simulink library "three_phase_voltage_with_frt_emulator"  (R2026a)
settings: Solver=VariableStepAuto
undefined symbols (not defined in the file): filters, frt_data, grid_emu, start_time_LVRT
libraries: $bdroot x6
settings Model: Creator=dbagn  LastModifiedBy=ltnbda

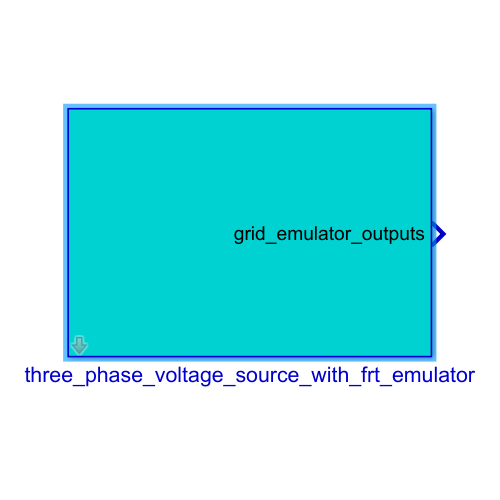
[thumbnail: Simulink's stored preview of the top-level diagram]
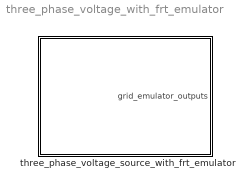
== system three_phase_voltage_with_frt_emulator ==
  three_phase_voltage_source_with_frt_emulator : Subsystem  mask{nominal_frequency_m=grid_emu.fgrid_nom, nominal_voltage_m=grid_emu.us_secondary_nom, Vemu_ref_norm_m=grid_emu.Vemu_ref_norm, vp_xi_pu_m=grid_emu.up_xi_pu_ref, vp_eta_pu_m=grid_emu.up_eta_pu_ref, vn_xi_pu_m=grid_emu.un_xi_pu_ref, vn_eta_pu_m=grid_emu.un_eta_pu, Am=filters.afe.SOF_50Hz.ss_c.A, Bm=filters.afe.SOF_50Hz.ss_c.B, Cm=filters.afe.SOF_50Hz.ss_c.C, enable_frt_1_m=frt_data.enable_frt_1, enable_frt_2_m=frt_data.enable_frt_2, start_time_LVRT_m=frt_data.start_time_LVRT, end_time_LVRT_m=frt_data.end_time_LVRT, deepPOSxi_m=frt_data.deepPOSxi, deepPOSeta_m=frt_data.deepPOSeta, deepNEGxi_m=frt_data.deepNEGxi, deepNEGeta_m=frt_data.deepNEGeta, Amplitude_U_m=frt_data.Amplitude_U, Amplitude_V_m=frt_data.Amplitude_V, Amplitude_W_m=frt_data.Amplitude_W, t_ramp_m=frt_data.t_ramp, Phase_shift_m=frt_data.Phase_shift}
      mask prompts: nominal_frequency_m "Nominal Frequency [Hz]"; nominal_voltage_m "Nominal Voltage [V]"; Vemu_ref_norm_m "Vemu_ref_norm"; vp_xi_pu_m "Vp_xi_pu [pu]"; vp_eta_pu_m "Vp_eta_pu [pu]"; vn_xi_pu_m "Vn_xi_pu [pu]"; vn_eta_pu_m "Vn_eta_pu [pu]"; Am "LVRT_flt_ss.A"; Bm "LVRT_flt_ss.B"; Cm "LVRT_flt_ss.C"; enable_frt_1_m "enable_frt_1"; enable_frt_2_m "enable_frt_2"; start_time_LVRT_m "Start_time_LVRT"; end_time_LVRT_m "End_time_LVRT"; deepPOSxi_m "deepPOSxi"; deepPOSeta_m "deepPOSeta"; deepNEGxi_m "deepNEGxi"; deepNEGeta_m "deepNEGeta"; Amplitude_U_m "Amplitude_U"; Amplitude_V_m "Amplitude_V"; Amplitude_W_m "Amplitude_W"; t_ramp_m "t_ramp"; Phase_shift_m "Phase_shift"

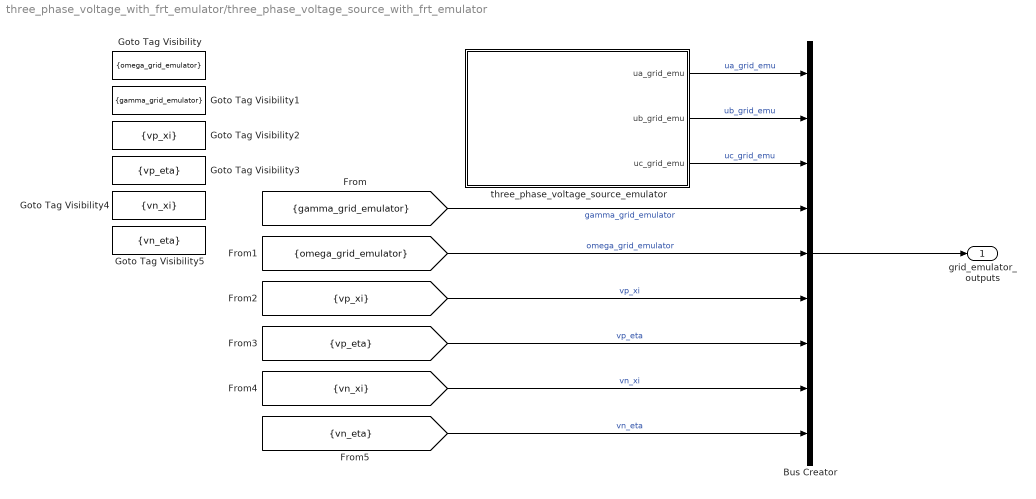
== system three_phase_voltage_with_frt_emulator/three_phase_voltage_source_with_frt_emulator ==
  Bus Creator : BusCreator  Inputs=9
  Goto Tag Visibility : GotoTagVisibility  GotoTag=omega_grid_emulator
  Goto Tag Visibility1 : GotoTagVisibility  GotoTag=gamma_grid_emulator
  Goto Tag Visibility2 : GotoTagVisibility  GotoTag=vp_xi
  Goto Tag Visibility3 : GotoTagVisibility  GotoTag=vp_eta
  Goto Tag Visibility4 : GotoTagVisibility  GotoTag=vn_xi
  Goto Tag Visibility5 : GotoTagVisibility  GotoTag=vn_eta
  three_phase_voltage_source_emulator : Subsystem
  grid_emulator_outputs : Outport  VectorParamsAs1DForOutWhenUnconnected=off
  wires:
  Bus Creator/1 -> grid_emulator_outputs/1
  three_phase_voltage_source_emulator/1(ua_grid_emu) -> Bus Creator/1  "ua_grid_emu"
  three_phase_voltage_source_emulator/2(ub_grid_emu) -> Bus Creator/2  "ub_grid_emu"
  three_phase_voltage_source_emulator/3(uc_grid_emu) -> Bus Creator/3  "uc_grid_emu"
  [omega_grid_emulator] -> Bus Creator/5  "omega_grid_emulator"
  [gamma_grid_emulator] -> Bus Creator/4  "gamma_grid_emulator"
  [vp_xi] -> Bus Creator/6  "vp_xi"
  [vp_eta] -> Bus Creator/7  "vp_eta"
  [vn_xi] -> Bus Creator/8  "vn_xi"
  [vn_eta] -> Bus Creator/9  "vn_eta"

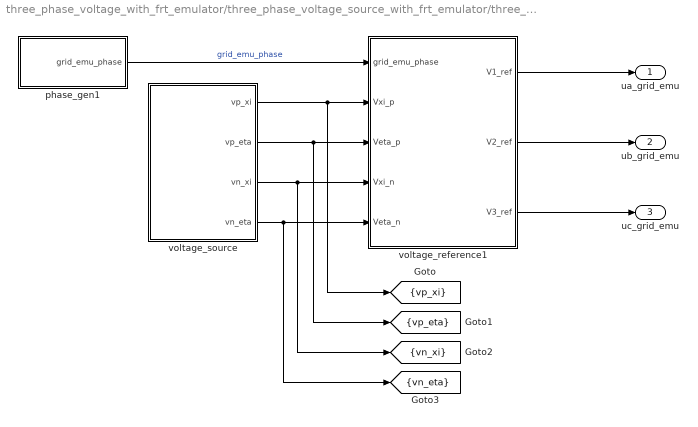
== system three_phase_voltage_with_frt_emulator/three_phase_voltage_source_with_frt_emulator/three_phase_voltage_source_emulator ==
  phase_gen1 : Subsystem
  voltage_reference1 : Subsystem
  voltage_source : Subsystem
  ua_grid_emu : Outport  VectorParamsAs1DForOutWhenUnconnected=off
  ub_grid_emu : Outport  Port=2  VectorParamsAs1DForOutWhenUnconnected=off
  uc_grid_emu : Outport  Port=3  VectorParamsAs1DForOutWhenUnconnected=off
  tag scope: vn_eta=scoped, vn_xi=scoped, vp_eta=scoped, vp_xi=scoped
  wires:
  voltage_reference1/2(V2_ref) -> ub_grid_emu/1
  voltage_reference1/3(V3_ref) -> uc_grid_emu/1
  voltage_source/3(vn_xi) -> [vn_xi], voltage_reference1/4(Vxi_n)
  voltage_source/1(vp_xi) -> [vp_xi], voltage_reference1/2(Vxi_p)
  voltage_source/4(vn_eta) -> [vn_eta], voltage_reference1/5(Veta_n)
  phase_gen1/1(grid_emu_phase) -> voltage_reference1/1(grid_emu_phase)  "grid_emu_phase"
  voltage_reference1/1(V1_ref) -> ua_grid_emu/1
  voltage_source/2(vp_eta) -> [vp_eta], voltage_reference1/3(Veta_p)

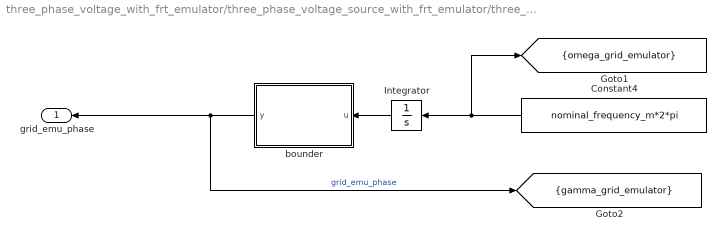
== system three_phase_voltage_with_frt_emulator/three_phase_voltage_source_with_frt_emulator/three_phase_voltage_source_emulator/phase_gen1 ==
  Constant4 : Constant  Value=nominal_frequency_m*2*pi
  Integrator : Integrator
  bounder : MATLAB Function  TreatAsAtomicUnit=on
  grid_emu_phase : Outport  VectorParamsAs1DForOutWhenUnconnected=off
  tag scope: gamma_grid_emulator=scoped, omega_grid_emulator=scoped
  wires:
  Integrator/1 -> bounder/1(u)
  Constant4/1 -> Integrator/1, [omega_grid_emulator]
  bounder/1(y) -> grid_emu_phase/1, [gamma_grid_emulator]  "grid_emu_phase"

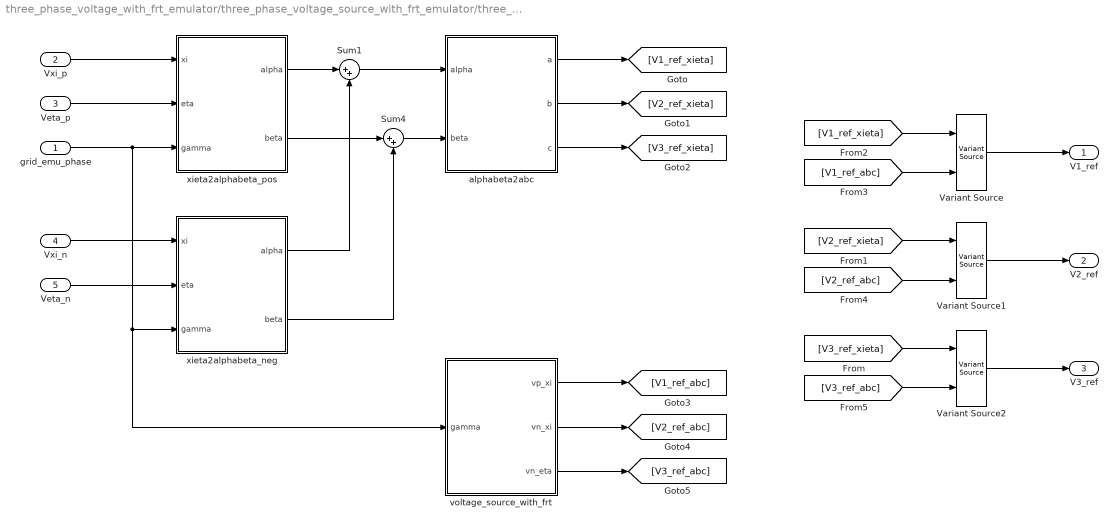
== system three_phase_voltage_with_frt_emulator/three_phase_voltage_source_with_frt_emulator/three_phase_voltage_source_emulator/voltage_reference1 ==
  grid_emu_phase : Inport
  Vxi_p : Inport  Port=2
  Veta_p : Inport  Port=3
  Vxi_n : Inport  Port=4
  Veta_n : Inport  Port=5
  Sum1 : Sum  Inputs=|++
  Sum4 : Sum  Inputs=|++
  Variant Source : VariantSource  VariantControls={(enable_frt_2_m || ~(enable_frt_1_m || enable_frt_1_m)) == 1, enable_frt_1_m == 1}
  Variant Source1 : VariantSource  VariantControls={(enable_frt_2_m || ~(enable_frt_1_m || enable_frt_1_m)) == 1, enable_frt_1_m == 1}
  Variant Source2 : VariantSource  VariantControls={(enable_frt_2_m || ~(enable_frt_1_m || enable_frt_1_m)) == 1, enable_frt_1_m == 1}
  alphabeta2abc : MATLAB Function  TreatAsAtomicUnit=on
  voltage_source_with_frt : Subsystem
  xieta2alphabeta_neg : MATLAB Function  TreatAsAtomicUnit=on
  xieta2alphabeta_pos : MATLAB Function  TreatAsAtomicUnit=on
  V1_ref : Outport  VectorParamsAs1DForOutWhenUnconnected=off
  V2_ref : Outport  Port=2  VectorParamsAs1DForOutWhenUnconnected=off
  V3_ref : Outport  Port=3  VectorParamsAs1DForOutWhenUnconnected=off
  wires:
  [V3_ref_xieta] -> Variant Source2/1
  [V3_ref_abc] -> Variant Source2/2
  Variant Source2/1 -> V3_ref/1
  [V2_ref_abc] -> Variant Source1/2
  [V2_ref_xieta] -> Variant Source1/1
  Variant Source1/1 -> V2_ref/1
  [V1_ref_abc] -> Variant Source/2
  [V1_ref_xieta] -> Variant Source/1
  voltage_source_with_frt/1(vp_xi) -> [V1_ref_abc]
  voltage_source_with_frt/2(vn_xi) -> [V2_ref_abc]
  voltage_source_with_frt/3(vn_eta) -> [V3_ref_abc]
  alphabeta2abc/3(c) -> [V3_ref_xieta]
  alphabeta2abc/2(b) -> [V2_ref_xieta]
  alphabeta2abc/1(a) -> [V1_ref_xieta]
  Variant Source/1 -> V1_ref/1
  Veta_n/1 -> xieta2alphabeta_neg/2(eta)
  Vxi_n/1 -> xieta2alphabeta_neg/1(xi)
  Veta_p/1 -> xieta2alphabeta_pos/2(eta)
  Vxi_p/1 -> xieta2alphabeta_pos/1(xi)
  grid_emu_phase/1 -> xieta2alphabeta_pos/3(gamma), xieta2alphabeta_neg/3(gamma), voltage_source_with_frt/1(gamma)
  xieta2alphabeta_neg/2(beta) -> Sum4/2
  xieta2alphabeta_neg/1(alpha) -> Sum1/2
  Sum4/1 -> alphabeta2abc/2(beta)
  xieta2alphabeta_pos/2(beta) -> Sum4/1
  Sum1/1 -> alphabeta2abc/1(alpha)
  xieta2alphabeta_pos/1(alpha) -> Sum1/1

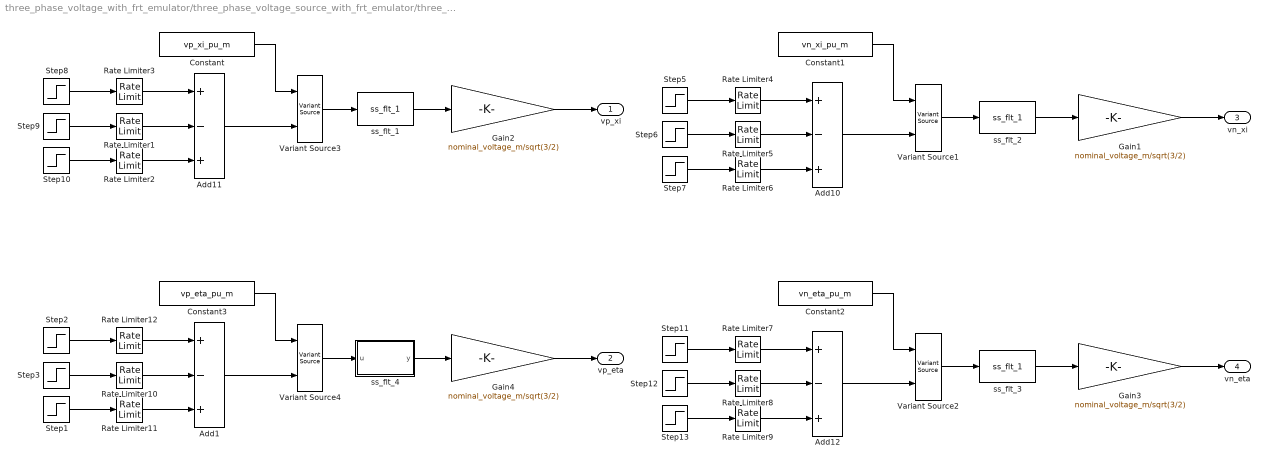
== system three_phase_voltage_with_frt_emulator/three_phase_voltage_source_with_frt_emulator/three_phase_voltage_source_emulator/voltage_source ==
  Add{1,10..12} (4 alike) : Sum  Inputs=+-+
  Constant : Constant  Value=vp_xi_pu_m
  Constant1 : Constant  Value=vn_xi_pu_m
  Constant2 : Constant  Value=vn_eta_pu_m
  Constant3 : Constant  Value=vp_eta_pu_m
  Gain{1..4} (4 alike) : Gain  Gain=nominal_voltage_m/sqrt(3/2)
  Rate Limiter{1..12} (12 alike) : RateLimiter  RisingSlewLimit=Vemu_ref_norm_m/t_ramp_m  FallingSlewLimit=-Vemu_ref_norm_m/t_ramp_m  SampleTimeMode=inherited
  Step1 : Step  Time=end_time_LVRT_m  FinalValue=deepPOSeta_m  SampleTime=0
  Step10 : Step  Time=end_time_LVRT_m  FinalValue=vp_xi_pu_m*deepPOSxi_m  SampleTime=0
  Step11 : Step  Time=0  FinalValue=vn_eta_pu_m  SampleTime=0
  Step12 : Step  Time=start_time_LVRT_m  FinalValue=deepNEGeta_m  SampleTime=0
  Step13 : Step  Time=end_time_LVRT_m  FinalValue=deepNEGeta_m  SampleTime=0
  Step2 : Step  Time=0  FinalValue=vp_eta_pu_m  SampleTime=0
  Step3 : Step  Time=start_time_LVRT_m  FinalValue=deepPOSeta_m  SampleTime=0
  Step5 : Step  Time=0  FinalValue=vn_xi_pu_m  SampleTime=0
  Step6 : Step  Time=start_time_LVRT_m  FinalValue=deepNEGxi_m  SampleTime=0
  Step7 : Step  Time=end_time_LVRT_m  FinalValue=deepNEGxi_m  SampleTime=0
  Step8 : Step  Time=0  FinalValue=vp_xi_pu_m  SampleTime=0
  Step9 : Step  Time=start_time_LVRT_m  FinalValue=vp_xi_pu_m*deepPOSxi_m  SampleTime=0
  Variant Source{1..4} (4 alike) : VariantSource  VariantControls={(enable_frt_1_m || enable_frt_2_m) == 0, (enable_frt_1_m || enable_frt_2_m) == 1}
  ss_flt_1 : $bdroot/three_phase_voltage_source_with_frt_emulator/three_phase_voltage_source_emulator/voltage_reference1/voltage_source_with_frt/ss_flt_1  SystemSampleTime=-1  VariantActivationTime=update diagram  EmptyChoice=off  PassThrough=off  PassThroughVariantControl=(default)  EmptyChoiceVariantControl=(default)  AllowFlexibleInterface=on  Latency=0  AutoFrameSizeCalculation=off
  ss_flt_2 : $bdroot/three_phase_voltage_source_with_frt_emulator/three_phase_voltage_source_emulator/voltage_reference1/voltage_source_with_frt/ss_flt_1  SystemSampleTime=-1  VariantActivationTime=update diagram  EmptyChoice=off  PassThrough=off  PassThroughVariantControl=(default)  EmptyChoiceVariantControl=(default)  AllowFlexibleInterface=on  Latency=0  AutoFrameSizeCalculation=off
  ss_flt_3 : $bdroot/three_phase_voltage_source_with_frt_emulator/three_phase_voltage_source_emulator/voltage_reference1/voltage_source_with_frt/ss_flt_1  SystemSampleTime=-1  VariantActivationTime=update diagram  EmptyChoice=off  PassThrough=off  PassThroughVariantControl=(default)  EmptyChoiceVariantControl=(default)  AllowFlexibleInterface=on  Latency=0  AutoFrameSizeCalculation=off
  ss_flt_4 : Subsystem
  vp_xi : Outport  VectorParamsAs1DForOutWhenUnconnected=off
  vp_eta : Outport  Port=2  VectorParamsAs1DForOutWhenUnconnected=off
  vn_xi : Outport  Port=3  VectorParamsAs1DForOutWhenUnconnected=off
  vn_eta : Outport  Port=4  VectorParamsAs1DForOutWhenUnconnected=off
  wires:
  ss_flt_3/1 -> Gain3/1
  ss_flt_2/1 -> Gain1/1
  Variant Source2/1 -> ss_flt_3/1
  Variant Source1/1 -> ss_flt_2/1
  ss_flt_1/1 -> Gain2/1
  Constant2/1 -> Variant Source2/1
  Add12/1 -> Variant Source2/2
  Constant1/1 -> Variant Source1/1
  Add10/1 -> Variant Source1/2
  Constant/1 -> Variant Source3/1
  Variant Source3/1 -> ss_flt_1/1
  Add11/1 -> Variant Source3/2
  Step13/1 -> Rate Limiter9/1
  Step10/1 -> Rate Limiter2/1
  Rate Limiter6/1 -> Add10/3
  Rate Limiter4/1 -> Add10/1
  Rate Limiter9/1 -> Add12/3
  Rate Limiter8/1 -> Add12/2
  Rate Limiter3/1 -> Add11/1
  Step9/1 -> Rate Limiter1/1
  Rate Limiter1/1 -> Add11/2
  Step11/1 -> Rate Limiter7/1
  Step12/1 -> Rate Limiter8/1
  Step8/1 -> Rate Limiter3/1
  Rate Limiter7/1 -> Add12/1
  Step5/1 -> Rate Limiter4/1
  Rate Limiter5/1 -> Add10/2
  Step6/1 -> Rate Limiter5/1
  Step7/1 -> Rate Limiter6/1
  Rate Limiter2/1 -> Add11/3
  Gain3/1 -> vn_eta/1
  Gain1/1 -> vn_xi/1
  Gain2/1 -> vp_xi/1
  Gain4/1 -> vp_eta/1
  Rate Limiter11/1 -> Add1/3
  Step2/1 -> Rate Limiter12/1
  Rate Limiter10/1 -> Add1/2
  Step3/1 -> Rate Limiter10/1
  Rate Limiter12/1 -> Add1/1
  Step1/1 -> Rate Limiter11/1
  Add1/1 -> Variant Source4/2
  Variant Source4/1 -> ss_flt_4/1(u)
  Constant3/1 -> Variant Source4/1
  ss_flt_4/1(y) -> Gain4/1

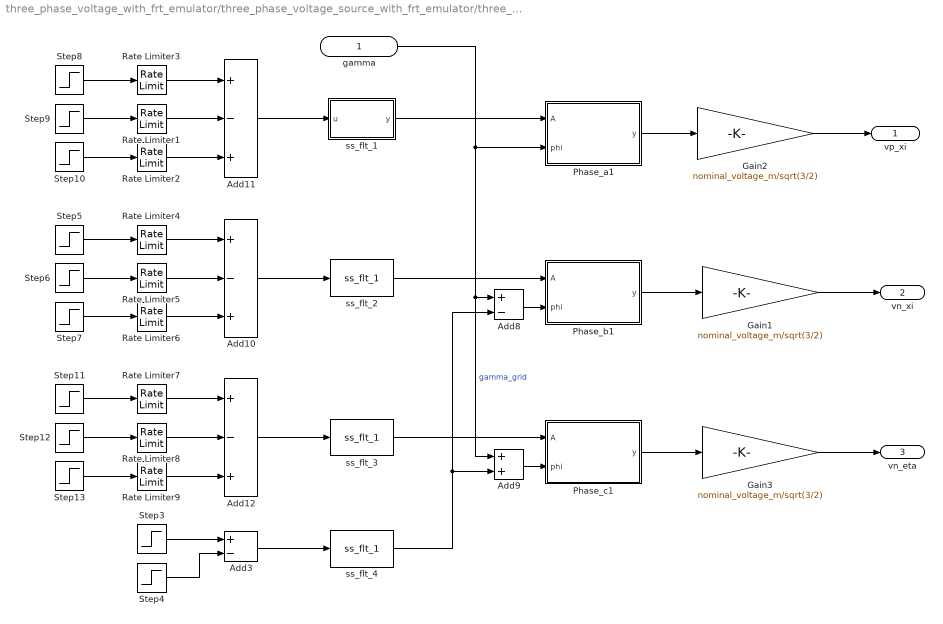
== system three_phase_voltage_with_frt_emulator/three_phase_voltage_source_with_frt_emulator/three_phase_voltage_source_emulator/voltage_reference1/voltage_source_with_frt ==
  gamma : Inport
  Add10 : Sum  Inputs=+-+
  Add11 : Sum  Inputs=+-+
  Add12 : Sum  Inputs=+-+
  Add3 : Sum  Inputs=+-
  Add8 : Sum  Inputs=+-
  Add9 : Sum
  Gain1 : Gain  Gain=nominal_voltage_m/sqrt(3/2)
  Gain2 : Gain  Gain=nominal_voltage_m/sqrt(3/2)
  Gain3 : Gain  Gain=nominal_voltage_m/sqrt(3/2)
  Phase_a1 : MATLAB Function  TreatAsAtomicUnit=on
  Phase_b1 : MATLAB Function  TreatAsAtomicUnit=on
  Phase_c1 : MATLAB Function  TreatAsAtomicUnit=on
  Rate Limiter{1..9} (9 alike) : RateLimiter  RisingSlewLimit=Vemu_ref_norm_m/t_ramp_m  FallingSlewLimit=-Vemu_ref_norm_m/t_ramp_m  SampleTimeMode=inherited
  Step10 : Step  Time=end_time_LVRT_m  FinalValue=Vemu_ref_norm_m*(1-Amplitude_U_m)  SampleTime=0
  Step11 : Step  Time=0  FinalValue=Vemu_ref_norm_m  SampleTime=0
  Step12 : Step  Time=start_time_LVRT_m  FinalValue=Vemu_ref_norm_m*(1-Amplitude_W_m)  SampleTime=0
  Step13 : Step  Time=end_time_LVRT_m  FinalValue=Vemu_ref_norm_m*(1-Amplitude_W_m)  SampleTime=0
  Step3 : Step  Time=start_time_LVRT  FinalValue=Phase_shift_m  SampleTime=0
  Step4 : Step  Time=end_time_LVRT_m  FinalValue=Phase_shift_m  SampleTime=0
  Step5 : Step  Time=0  FinalValue=Vemu_ref_norm_m  SampleTime=0
  Step6 : Step  Time=start_time_LVRT_m  FinalValue=Vemu_ref_norm_m*(1-Amplitude_V_m)  SampleTime=0
  Step7 : Step  Time=end_time_LVRT_m  FinalValue=Vemu_ref_norm_m*(1-Amplitude_V_m)  SampleTime=0
  Step8 : Step  Time=0  FinalValue=Vemu_ref_norm_m  SampleTime=0
  Step9 : Step  Time=start_time_LVRT_m  FinalValue=Vemu_ref_norm_m*(1-Amplitude_U_m)  SampleTime=0
  ss_flt_1 : Subsystem
  ss_flt_2 : $bdroot/three_phase_voltage_source_with_frt_emulator/three_phase_voltage_source_emulator/voltage_reference1/voltage_source_with_frt/ss_flt_1  SystemSampleTime=-1  VariantActivationTime=update diagram  EmptyChoice=off  PassThrough=off  PassThroughVariantControl=(default)  EmptyChoiceVariantControl=(default)  AllowFlexibleInterface=on  Latency=0  AutoFrameSizeCalculation=off
  ss_flt_3 : $bdroot/three_phase_voltage_source_with_frt_emulator/three_phase_voltage_source_emulator/voltage_reference1/voltage_source_with_frt/ss_flt_1  SystemSampleTime=-1  VariantActivationTime=update diagram  EmptyChoice=off  PassThrough=off  PassThroughVariantControl=(default)  EmptyChoiceVariantControl=(default)  AllowFlexibleInterface=on  Latency=0  AutoFrameSizeCalculation=off
  ss_flt_4 : $bdroot/three_phase_voltage_source_with_frt_emulator/three_phase_voltage_source_emulator/voltage_reference1/voltage_source_with_frt/ss_flt_1  SystemSampleTime=-1  VariantActivationTime=update diagram  EmptyChoice=off  PassThrough=off  PassThroughVariantControl=(default)  EmptyChoiceVariantControl=(default)  AllowFlexibleInterface=on  Latency=0  AutoFrameSizeCalculation=off
  vp_xi : Outport  VectorParamsAs1DForOutWhenUnconnected=off
  vn_xi : Outport  Port=2  VectorParamsAs1DForOutWhenUnconnected=off
  vn_eta : Outport  Port=3  VectorParamsAs1DForOutWhenUnconnected=off
  wires:
  Gain3/1 -> vn_eta/1
  Gain1/1 -> vn_xi/1
  Gain2/1 -> vp_xi/1
  Add3/1 -> ss_flt_4/1
  Step4/1 -> Add3/2
  Step3/1 -> Add3/1
  Phase_c1/1(y) -> Gain3/1
  Phase_b1/1(y) -> Gain1/1
  Phase_a1/1(y) -> Gain2/1
  Rate Limiter7/1 -> Add12/1
  Step11/1 -> Rate Limiter7/1
  Rate Limiter9/1 -> Add12/3
  Step13/1 -> Rate Limiter9/1
  Rate Limiter8/1 -> Add12/2
  Step12/1 -> Rate Limiter8/1
  Rate Limiter6/1 -> Add10/3
  Rate Limiter5/1 -> Add10/2
  Rate Limiter4/1 -> Add10/1
  Rate Limiter2/1 -> Add11/3
  Rate Limiter1/1 -> Add11/2
  Rate Limiter3/1 -> Add11/1
  Add11/1 -> ss_flt_1/1(u)
  Step10/1 -> Rate Limiter2/1
  Step9/1 -> Rate Limiter1/1
  Step8/1 -> Rate Limiter3/1
  Step7/1 -> Rate Limiter6/1
  Step6/1 -> Rate Limiter5/1
  Step5/1 -> Rate Limiter4/1
  Add10/1 -> ss_flt_2/1
  Add8/1 -> Phase_b1/2(phi)
  Add9/1 -> Phase_c1/2(phi)
  gamma/1 -> Phase_a1/2(phi), Add8/1, Add9/1  "gamma_grid"
  Add12/1 -> ss_flt_3/1
  ss_flt_1/1(y) -> Phase_a1/1(A)
  ss_flt_2/1 -> Phase_b1/1(A)
  ss_flt_3/1 -> Phase_c1/1(A)
  ss_flt_4/1 -> Add8/2, Add9/2

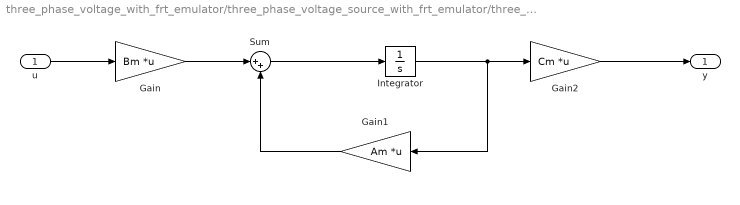
== system three_phase_voltage_with_frt_emulator/three_phase_voltage_source_with_frt_emulator/three_phase_voltage_source_emulator/voltage_source/ss_flt_4 ==
  u : Inport
  Gain : Gain  Gain=Bm  Multiplication=Matrix(K*u)
  Gain1 : Gain  Gain=Am  Multiplication=Matrix(K*u)
  Gain2 : Gain  Gain=Cm  Multiplication=Matrix(K*u)
  Integrator : Integrator
  Sum : Sum  Inputs=|++
  y : Outport
  wires:
  Gain/1 -> Sum/1
  Sum/1 -> Integrator/1
  u/1 -> Gain/1
  Integrator/1 -> Gain1/1, Gain2/1
  Gain1/1 -> Sum/2
  Gain2/1 -> y/1

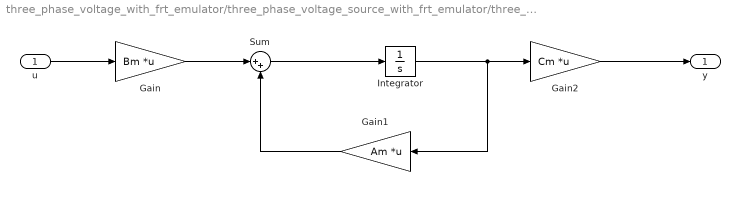
== system three_phase_voltage_with_frt_emulator/three_phase_voltage_source_with_frt_emulator/three_phase_voltage_source_emulator/voltage_reference1/voltage_source_with_frt/ss_flt_1 ==
  u : Inport
  Gain : Gain  Gain=Bm  Multiplication=Matrix(K*u)
  Gain1 : Gain  Gain=Am  Multiplication=Matrix(K*u)
  Gain2 : Gain  Gain=Cm  Multiplication=Matrix(K*u)
  Integrator : Integrator
  Sum : Sum  Inputs=|++
  y : Outport
  wires:
  Gain/1 -> Sum/1
  Sum/1 -> Integrator/1
  u/1 -> Gain/1
  Integrator/1 -> Gain1/1, Gain2/1
  Gain1/1 -> Sum/2
  Gain2/1 -> y/1

== matlab function three_phase_voltage_with_frt_emulator/three_phase_voltage_source_with_frt_emulator/three_phase_voltage_source_emulator/phase_gen1/bounder ==
  data: u input; y output
function y = bounder(u)    
    y = -pi + mod(u+3*pi,2*pi);
end

== matlab function three_phase_voltage_with_frt_emulator/three_phase_voltage_source_with_frt_emulator/three_phase_voltage_source_emulator/voltage_reference1/alphabeta2abc ==
  data: alpha input; a output; beta input; b output; c output
function [a,b,c] = alphabeta2abc(alpha,beta)

    a  =  alpha;
    b  =  -0.5*alpha + sqrt(3)/2*beta;
    c  =  -0.5*alpha - sqrt(3)/2*beta;
end

== matlab function three_phase_voltage_with_frt_emulator/three_phase_voltage_source_with_frt_emulator/three_phase_voltage_source_emulator/voltage_reference1/voltage_source_with_frt/Phase_a1 ==
  data: A input; y output; phi input
function y = Phase_a(A,phi)

    y = A*cos(phi);

end

== matlab function three_phase_voltage_with_frt_emulator/three_phase_voltage_source_with_frt_emulator/three_phase_voltage_source_emulator/voltage_reference1/voltage_source_with_frt/Phase_b1 ==
  data: A input; y output; phi input
function y = Phase_b(A,phi)

    y = A*cos(phi-2*pi/3);

end

== matlab function three_phase_voltage_with_frt_emulator/three_phase_voltage_source_with_frt_emulator/three_phase_voltage_source_emulator/voltage_reference1/voltage_source_with_frt/Phase_c1 ==
  data: A input; y output; phi input
function y = Phase_c(A,phi)

    y = A*cos(phi-4*pi/3);

end

== matlab function three_phase_voltage_with_frt_emulator/three_phase_voltage_source_with_frt_emulator/three_phase_voltage_source_emulator/voltage_reference1/xieta2alphabeta_neg ==
  data: xi input; alpha output; eta input; gamma input; beta output
function [alpha,beta] = xieta2alphabeta_neg(xi,eta,gamma)

    alpha  =  xi*cos(gamma) + eta*sin(gamma);
    beta = -xi*sin(gamma) + eta*cos(gamma);

end

== matlab function three_phase_voltage_with_frt_emulator/three_phase_voltage_source_with_frt_emulator/three_phase_voltage_source_emulator/voltage_reference1/xieta2alphabeta_pos ==
  data: xi input; alpha output; eta input; gamma input; beta output
function [alpha,beta] = xieta2alphabeta_pos(xi,eta,gamma)

    alpha  =  xi*cos(gamma) - eta*sin(gamma);
    beta = xi*sin(gamma) + eta*cos(gamma);

end
